simulink model "pendulum"  (Simulink 9.0)
settings: Solver=FixedStepAuto  StartTime=0.0  StopTime=20  FixedStep=0.001  MaxStep=0.01  RelTol=1e-3
values from neighbouring files (symbols this model uses):
  Ts = 1/250    (= 0.004)    [IdealParameter.m]    (also in ParLuk11.m = 0.05; Parameter.m = 0.03; ParameterIdeal.m; ParameterVIVE.m)
undefined symbols (not defined in the file or in its folder): DiscIntNeverNeededParam
libraries: simulink x1
settings Model: Creator=Jan  LastModifiedBy=Jan
settings DataIOCC: SaveFormat=Dataset
settings OptimizationCC: LifeSpan=auto
settings DebuggingCC: UnderspecifiedInitializationDetection=Simplified  MergeDetectMultiDrivingBlocksExec=error  SFUnexpectedBacktrackingDiag=error  SFNoUnconditionalDefaultTransitionDiag=error  SFExecutionAtInitializationDiag=warning
settings HardwareCC: ProdBitPerPointer=64  ProdBitPerSizeT=64  ProdBitPerPtrDiffT=64  ProdLargestAtomicFloat=Float  ProdIntDivRoundTo=Zero  ProdEndianess=LittleEndian  ProdWordSize=64  ProdHWDeviceType=Intel->x86-64 (Windows64)
settings ModelReferenceCC: PropagateSignalLabelsOutOfModel=on
settings CodeAppCC: StateflowObjectComments=off
settings GRTTargetCC: TargetLangStandard=C99 (ISO)
settings ConfigComp: CovMetricSettings=dwe  CovHtmlReporting=off  CovSaveCumulativeToWorkspaceVar=off  CovSaveSingleToWorkspaceVar=off  CovExternalEMLEnable=on

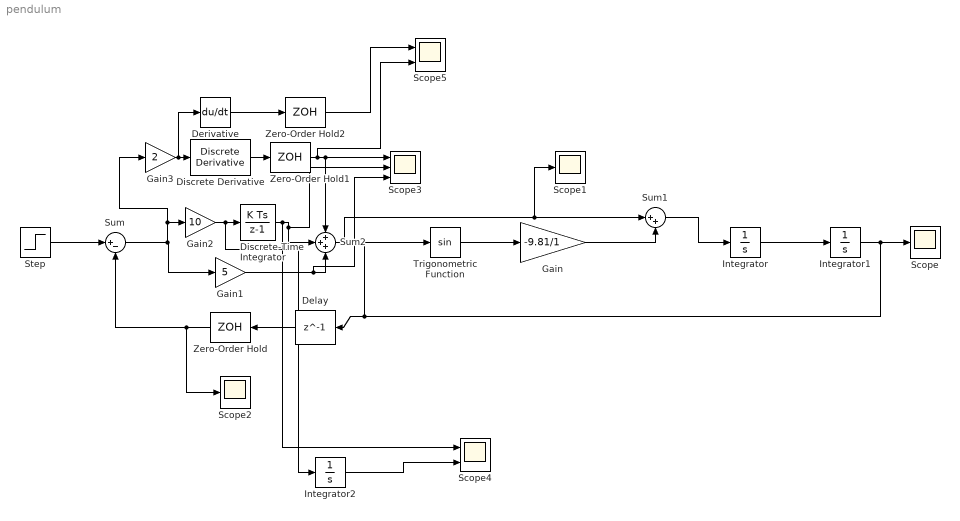
== system pendulum ==
  Delay : Delay  DelayLength=1  InitialCondition=pi/3  SampleTime=Ts
  Derivative : Derivative  CoefficientInTFapproximation=Ts
  Discrete Derivative : simulink/Discrete/Discrete Derivative  gainval=1.0  ICPrevScaledInput=0.0  OutMin=[]  OutMax=[]  OutDataType=fixdt(1, 16)  OutScaling=2^-10  DoSatur=off
  Discrete-Time Integrator : DiscreteIntegrator  InitialConditionSetting=State (most efficient)  SampleTime=Ts  ICPrevOutput=DiscIntNeverNeededParam  ICPrevScaledInput=DiscIntNeverNeededParam
  Gain : Gain  Gain=-9.81/1
  Gain1 : Gain  Gain=5
  Gain2 : Gain  Gain=10
  Gain3 : Gain  Gain=2
  Integrator : Integrator
  Integrator1 : Integrator  InitialCondition=pi/3
  Integrator2 : Integrator
  Scope : Scope
  Scope1 : Scope
  Scope2 : Scope
  Scope3 : Scope  NumInputPorts=3
  Scope4 : Scope  NumInputPorts=2
  Scope5 : Scope  NumInputPorts=2
  Step : Step  Time=0  After=0  SampleTime=0
  Sum : Sum  Inputs=|+-
  Sum1 : Sum  Inputs=|++
  Sum2 : Sum  Inputs=+++
  Trigonometric Function : Trigonometry
  Zero-Order Hold : ZeroOrderHold  SampleTime=Ts
  Zero-Order Hold1 : ZeroOrderHold  SampleTime=Ts
  Zero-Order Hold2 : ZeroOrderHold  SampleTime=Ts
  wires:
  Gain/1 -> Sum1/2
  Integrator/1 -> Integrator1/1
  Integrator1/1 -> Scope/1, Delay/1, Trigonometric Function/1
  Trigonometric Function/1 -> Gain/1
  Step/1 -> Sum/1
  Sum1/1 -> Integrator/1
  Sum2/1 -> Scope1/1, Sum1/1
  Sum/1 -> Gain3/1, Gain2/1, Gain1/1
  Gain1/1 -> Scope3/3, Sum2/3
  Discrete-Time Integrator/1 -> Scope4/1, Scope3/2, Sum2/2
  Gain2/1 -> Integrator2/1, Discrete-Time Integrator/1
  Zero-Order Hold1/1 -> Scope5/2, Scope3/1, Sum2/1
  Gain3/1 -> Derivative/1, Discrete Derivative/1
  Zero-Order Hold/1 -> Scope2/1, Sum/2
  Discrete Derivative/1 -> Zero-Order Hold1/1
  Integrator2/1 -> Scope4/2
  Derivative/1 -> Zero-Order Hold2/1
  Zero-Order Hold2/1 -> Scope5/1
  Delay/1 -> Zero-Order Hold/1
